simulink model "LQR_LQG_Inverted_Pendulum_a"  (R2023a)
settings: Solver=ode4  StartTime=0.0  StopTime=10.0  RelTol=1e-3
undefined symbols (not defined in the file or in its folder): A, A_kf, B, B_kf, C, C_kf, D_kf, K, x0, xhat0
settings Model: Creator=ASUS  LastModifiedBy=Thu

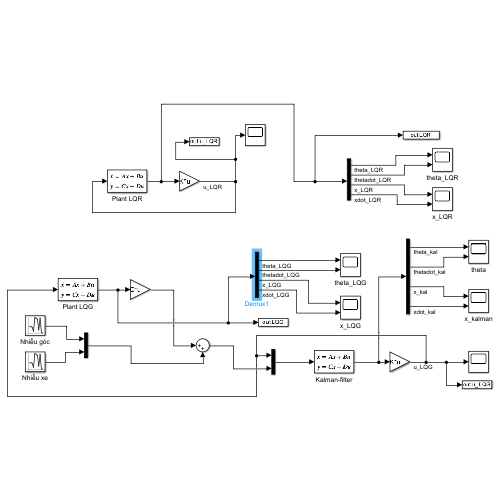
[thumbnail: Simulink's stored preview of the top-level diagram]
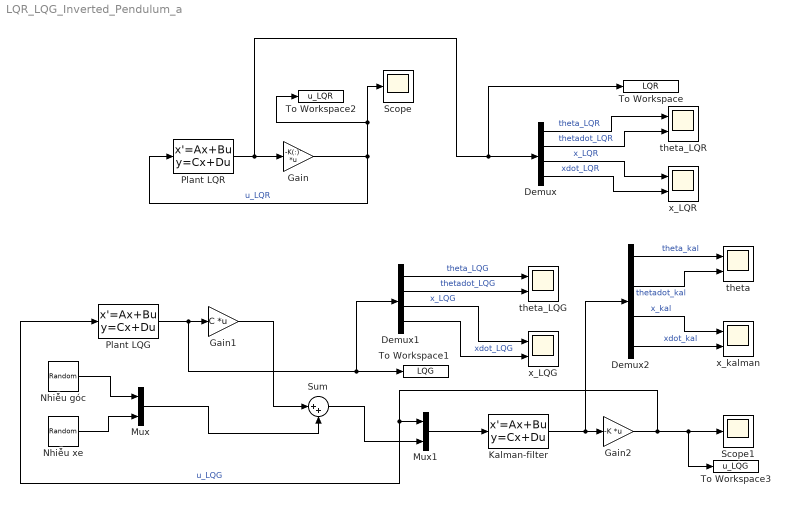
== system LQR_LQG_Inverted_Pendulum_a ==
  Demux : Demux
  Demux1 : Demux
  Demux2 : Demux
  Gain : Gain  Gain=-K(:)'  Multiplication=Matrix(K*u)
  Gain1 : Gain  Gain=C  Multiplication=Matrix(K*u)
  Gain2 : Gain  Gain=-K  Multiplication=Matrix(K*u)
  Kalman-filter : StateSpace  A=A_kf  B=B_kf  C=C_kf  D=D_kf  InitialCondition=xhat0
  Mux : Mux  Inputs=2
  Mux1 : Mux  Inputs=2
  Nhiễu góc : RandomNumber  Variance=0.001  SampleTime=0.001
  Nhiễu xe : RandomNumber  Variance=0.01  SampleTime=0.001
  Plant LQG : StateSpace  A=A  B=B  C=eye(4)  D=zeros(4,1)  InitialCondition=x0
  Plant LQR : StateSpace  A=A  B=B  C=eye(4)  D=zeros(4,1)  InitialCondition=x0
  Scope : Scope
  Scope1 : Scope
  Sum : Sum  Inputs=|++
  To Workspace : ToWorkspace  VariableName=LQR  SaveFormat=Timeseries  SampleTime=-1
  To Workspace1 : ToWorkspace  VariableName=LQG  SaveFormat=Timeseries  SampleTime=-1
  To Workspace2 : ToWorkspace  VariableName=u_LQR  SaveFormat=Timeseries  SampleTime=-1
  To Workspace3 : ToWorkspace  VariableName=u_LQG  SaveFormat=Timeseries  SampleTime=-1
  theta : Scope  NumInputPorts=2
  theta_LQG : Scope  NumInputPorts=2
  theta_LQR : Scope  NumInputPorts=2
  x_LQG : Scope  NumInputPorts=2
  x_LQR : Scope  NumInputPorts=2
  x_kalman : Scope  NumInputPorts=2
  wires:
  Plant LQR/1 -> To Workspace/1, Demux/1, Gain/1
  Gain/1 -> To Workspace2/1, Scope/1, Plant LQR/1  "u_LQR"
  Plant LQG/1 -> Demux1/1, To Workspace1/1, Gain1/1
  Nhiễu xe/1 -> Mux/2
  Nhiễu góc/1 -> Mux/1
  Gain1/1 -> Sum/1
  Mux/1 -> Sum/2
  Kalman-filter/1 -> Demux2/1, Gain2/1
  Mux1/1 -> Kalman-filter/1
  Gain2/1 -> To Workspace3/1, Scope1/1, Plant LQG/1, Mux1/1  "u_LQG"
  Sum/1 -> Mux1/2
  Demux/3 -> x_LQR/1  "x_LQR"
  Demux/4 -> x_LQR/2  "xdot_LQR"
  Demux/1 -> theta_LQR/1  "theta_LQR"
  Demux/2 -> theta_LQR/2  "thetadot_LQR"
  Demux1/1 -> theta_LQG/1  "theta_LQG"
  Demux1/2 -> theta_LQG/2  "thetadot_LQG"
  Demux1/3 -> x_LQG/1  "x_LQG"
  Demux1/4 -> x_LQG/2  "xdot_LQG"
  Demux2/1 -> theta/1  "theta_kal"
  Demux2/2 -> theta/2  "thetadot_kal"
  Demux2/3 -> x_kalman/1  "x_kal"
  Demux2/4 -> x_kalman/2  "xdot_kal"
